simulink model "ETE_2004037"  (R2022b)
settings: Solver=VariableStepAuto  StartTime=0.0  StopTime=10.0  RelTol=1e-3
libraries: commrandsrc3 x1, dsparch4 x1
settings Model: Creator=Asus  LastModifiedBy=Asus

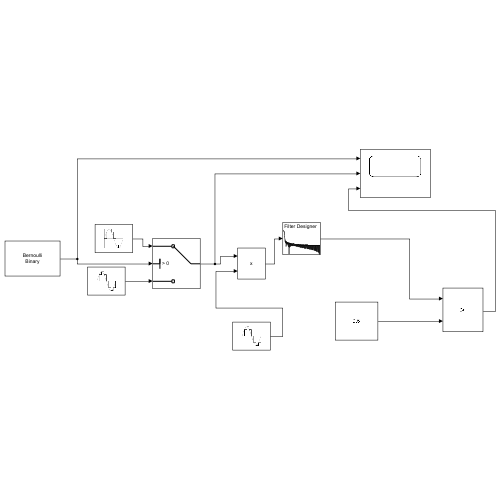
[thumbnail: Simulink's stored preview of the top-level diagram]
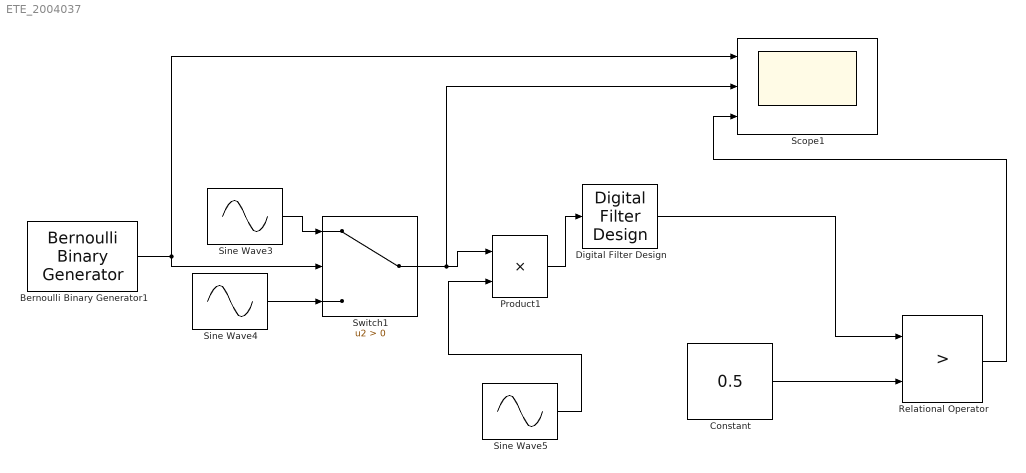
== system ETE_2004037 ==
  Bernoulli Binary Generator1 : commrandsrc3/Bernoulli Binary Generator  ProbabilityOfZero=0.5  SeedSource=Auto  Seed=0  SampleTime=1  SamplesPerFrame=1  OutputDataType=double  SimulateUsing=Interpreted execution
  Constant : Constant  Value=0.5
  Digital Filter Design : dsparch4/Digital Filter Design  mwdsp_browser_bugfix_var=off
  Product1 : Product
  Relational Operator : RelationalOperator  Operator=>  OutDataTypeStr=boolean  RndMeth=Simplest  InputSameDT=off
  Scope1 : Scope  NumInputPorts=3
  Sine Wave3 : Sin  Amplitude=2  Frequency=4*pi  SampleTime=0.01
  Sine Wave4 : Sin  Amplitude=0.5  Frequency=4*pi  SampleTime=0.01
  Sine Wave5 : Sin  Frequency=4*pi  SampleTime=0.01
  Switch1 : Switch  Criteria=u2 > Threshold  SaturateOnIntegerOverflow=off  InputSameDT=off
  wires:
  Constant/1 -> Relational Operator/2
  Relational Operator/1 -> Scope1/3
  Sine Wave4/1 -> Switch1/3
  Switch1/1 -> Product1/1, Scope1/2
  Bernoulli Binary Generator1/1 -> Switch1/2, Scope1/1
  Digital Filter Design/1 -> Relational Operator/1
  Sine Wave5/1 -> Product1/2
  Product1/1 -> Digital Filter Design/1
  Sine Wave3/1 -> Switch1/1
